simulink model "Check"  (R2019a)
settings: Solver=VariableStepAuto  StartTime=0.0  StopTime=10.0  RelTol=1e-3
settings Model: Creator=anton  LastModifiedBy=anton

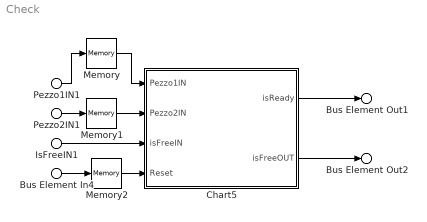
== system Check ==
  Pezzo1IN1 : Inport  PortName=Pezzo1IN
  Pezzo2IN1 : Inport  Port=2  PortName=Pezzo2IN
  IsFreeIN1 : Inport  Port=3  PortName=IsFreeIN
  Bus Element In4 : Inport  Port=4  PortName=Reset
  Chart5 : Stateflow chart  BlockKeywords=__PRM__SERIALIZED__DATA__:Stateflow Chart,Stateflow Diagram  TreatAsAtomicUnit=on
  Memory : Memory
  Memory1 : Memory
  Memory2 : Memory
  Bus Element Out1 : Outport  PortName=IsReady
  Bus Element Out2 : Outport  Port=2  PortName=IsFreeOUT
  wires:
  Chart5/1(isReady) -> Bus Element Out1/1
  IsFreeIN1/1 -> Chart5/3(isFreeIN)
  Chart5/2(isFreeOUT) -> Bus Element Out2/1
  Memory/1 -> Chart5/1(Pezzo1IN)
  Pezzo1IN1/1 -> Memory/1
  Pezzo2IN1/1 -> Memory1/1
  Memory1/1 -> Chart5/2(Pezzo2IN)
  Memory2/1 -> Chart5/4(Reset)
  Bus Element In4/1 -> Memory2/1

== stateflow chart Check/Chart5 ==
  state Idle
  state Pezzo1Available
  state Pezzo2Available
  state Check
    isReady = 1;
    isFreeOUT = 1;
  (default) -> Idle
  Check -> Idle : [Reset==1]
  Idle -> Pezzo1Available : [Pezzo1IN==1]
  Pezzo1Available -> Pezzo2Available : [Pezzo2IN==1]
  Pezzo2Available -> Check : [isFreeIN == 1]
  data: isReady output; isFreeOUT output; Pezzo1IN input; Pezzo2IN input; isFreeIN input; Reset input
